simulink model "Lure_Preisach"  (R2017b)
settings: Solver=FixedStepAuto  StartTime=0.0  StopTime=simTotalTime  FixedStep=0.05  MaxStep=0.1  MinStep=0.01  RelTol=1e-3
undefined symbols (not defined in the file): gridArea, gridDen, gridLength, hysteronMax, hysteronMin, initialRelays, inputFactor, inputMax, inputMin, offset, outputFactor, outputMax, outputMin, weightFunc, xyGrid
libraries: simulink x2
settings Model: Creator=Marco  LastModifiedBy=M. Vasquez Beltran

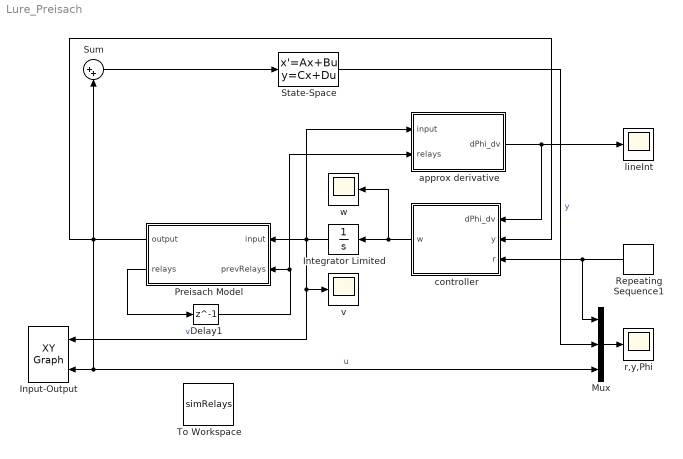
== system Lure_Preisach ==
  Delay1 : Delay  DelayLength=1  InitialCondition=initialRelays
  Input-Output : simulink/Sinks/XY Graph  xmin=inputMin*inputFactor  xmax=inputMax*inputFactor  ymin=outputMin*outputFactor  ymax=outputMax*outputFactor  st=-1
  Integrator Limited : Integrator  InitialCondition=0.75  UpperSaturationLimit=inputMax*0.99  LowerSaturationLimit=inputMin*0.99
  Mux : Mux  Inputs=3
  Preisach Model : MATLAB Function  TreatAsAtomicUnit=on
  Repeating Sequence1 : simulink/Sources/Repeating Sequence  rep_seq_t=sequenceTime  rep_seq_y=sequenceVal
  State-Space : StateSpace  A=-1  D=0  InitialCondition=-1.2
  Sum : Sum  Inputs=|++
  To Workspace : ToWorkspace  VariableName=simRelays  SampleTime=-1
  approx derivative : MATLAB Function  TreatAsAtomicUnit=on
  controller : MATLAB Function  TreatAsAtomicUnit=on
  lineInt : Scope
  r,y,Phi : Scope
  v : Scope
  w : Scope
  wires:
  Preisach Model/2(relays) -> Delay1/1
  Delay1/1 -> approx derivative/2(relays), Preisach Model/2(prevRelays)
  Sum/1 -> State-Space/1
  Preisach Model/1(output) -> controller/2(y), Sum/2, Input-Output/2, Mux/3  "u"
  State-Space/1 -> Mux/2  "y"
  Integrator Limited/1 -> approx derivative/1(input), Preisach Model/1(input), Input-Output/1, v/1  "v"
  approx derivative/1(dPhi_dv) -> controller/1(dPhi_dv), lineInt/1
  Repeating Sequence1/1 -> controller/3(r), Mux/1
  controller/1(w) -> Integrator Limited/1, w/1
  Mux/1 -> r,y,Phi/1

== matlab function Lure_Preisach/Preisach Model ==
  data: input input; prevRelays input; output output; weightFunc parameter; relays output; offset parameter; hysteronMin parameter; hysteronMax parameter; gridDen parameter; xyGrid parameter; gridLength parameter; gridArea parameter
function [output, relays] = fcn(input, prevRelays, ...
    weightFunc, offset, hysteronMin, hysteronMax, gridDen, xyGrid, gridLength, gridArea)

%     output = offset;
%     relays = prevRelays;
%     for i=1:gridDen
%         ii = gridDen-i+1; %index inversion for rows
%         for j=1:i
%             if( input >= xyGrid(i) && relays(ii,j) ~= hysteronMax )
%                 relays(ii,j) = hysteronMax;
%             elseif( input <= xyGrid(j) && relays(ii,j) ~= hysteronMin )
%                 relays(ii,j) = hysteronMin;
%             end
%             output = output + relays(ii,j)*weightFunc(ii,j)*gridArea;
%         end
%     end



%     relays = prevRelays;
%     for row=1:gridDen+1
%         if( row == gridDen+1 || input <= xyGrid(row) )
%             row = row-1;
%             irow = gridDen-row+1;
%             relays(irow:end, 1:row) = hysteronMax*fliplr(triu(ones(row, row)));
%             break;
%         end
%     end
%     for col=gridDen:-1:0
%         if( col == 0 || input >= xyGrid(col) )
%             col = col+1;
%             irow = gridDen-col+1;
%             relays(1:irow, col:end) = hysteronMin*fliplr(triu(ones(irow, irow)));
%             break;
%         end
%     end
%     output = sum(sum(relays(:,:).*weightFunc(:,:)))*gridArea + offset;



    relays = prevRelays;
    if( xyGrid(end) <= input )
        relays(:,:) = hysteronMax*fliplr(triu(ones(gridDen, gridDen)));
    elseif( input < xyGrid(1) )
        relays(:,:) = hysteronMin*fliplr(triu(ones(gridDen, gridDen)));
    else
        idx0 = 1;
        while( idx0 <= gridDen-1 )
            if( xyGrid(idx0) <= input && input < xyGrid(idx0+1) )
                col = idx0;
                row = gridDen-idx0+1;

                relays(row:end, 1:col) = hysteronMax*fliplr(triu(ones(col, col)));
                relays(1:row-1, col+1:end) = hysteronMin*fliplr(triu(ones(row-1, row-1)));
                break;
            end
            idx0 = idx0 + 1;
        end
    end
    output = sum(sum(relays(:,:).*weightFunc(:,:)))*gridArea + offset;

== matlab function Lure_Preisach/approx derivative ==
  data: input input; relays input; weightFunc parameter; hysteronMin parameter; hysteronMax parameter; offset parameter; gridDen parameter; dPhi_dv output; xyGrid parameter; gridLength parameter
function dPhi_dv = fcn(input, relays,...
     weightFunc, hysteronMin, hysteronMax, offset, gridDen, xyGrid, gridLength)

dPhi_dv = [0; 0];
if( xyGrid(end) <= input )
    return;
elseif( input < xyGrid(1) )
    return;
else
    idx0 = 1;
    while( idx0 <= gridDen-1 )
        if( xyGrid(idx0) <= input && input < xyGrid(idx0+1) )
            col = idx0;
            row = gridDen-idx0+1;
            
            for var=col:-1:1
                if( relays(row-1,var)==hysteronMin )
                    dPhi_dv(1) = dPhi_dv(1) + gridLength*weightFunc(row-1,var);
                end
            end
            
            for var=row:-1:1
                if( relays(var,col)==hysteronMax )
                    dPhi_dv(2) = dPhi_dv(2) + gridLength*weightFunc(var,col);
                end
            end
            
            break;
        end
        idx0 = idx0 + 1;
    end
end
dPhi_dv = 2*dPhi_dv;

end

== matlab function Lure_Preisach/controller ==
  data: dPhi_dv input; w output; y input; r input
function w    = fcn(dPhi_dv, y, r)

    k = 2;
    lineIntTh = 0.1;
    
%     if( abs(dPhi_dv(1)) <= lineIntTh && abs(dPhi_dv(2)) <= lineIntTh )
%         w = 0;
%     elseif( abs(dPhi_dv(1)) >= abs(dPhi_dv(2)) )
%         w = k*(r-y)/dPhi_dv(1);
%     else
%         w = -k*(r-y)/dPhi_dv(2);
%     end
    
%     w = 0;
%     signVec = dPhi_dv;
%     signVec(signVec>=0) = 1;
%     signVec(signVec<0) = -1;
%     if( abs(dPhi_dv(1)) > abs(dPhi_dv(2)) )
%         lambda = signVec(1)*max(abs([dPhi_dv(1), lineIntTh]));
%     else
%         lambda = signVec(2)*max(abs([dPhi_dv(2), lineIntTh]));
%     end
%     w = k*(r-y)/lambda;
    
    w = 0;
    if( r-y>0 )
        lambda = max(abs([dPhi_dv(1), lineIntTh]));
    else
        lambda = max(abs([dPhi_dv(2), lineIntTh]));
    end
    w = k*(r-y)/lambda;
    
%     w = 0;
%     e = r-y;
%     if ( e>0 )
%         if ( dPhi_dv(1)>0 )
%             w =  abs(e)/max(abs([lineIntTh, dPhi_dv(1)]));
%         elseif ( dPhi_dv(2)<0 )
%             w = -abs(e)/max(abs([lineIntTh, dPhi_dv(2)]));
%         elseif ( dPhi_dv(1)<=0 )
%             w = -abs(e)/max(abs([lineIntTh, dPhi_dv(2)]));
%         end
%     elseif( e<0 )
%         if ( dPhi_dv(2)>0 )
%             w = -abs(e)/max(abs([lineIntTh, dPhi_dv(2)]));
%         elseif ( dPhi_dv(1)<0 )
%             w =  abs(e)/max(abs([lineIntTh, dPhi_dv(1)]));
%         elseif ( dPhi_dv(2)<=0 )
%             w = abs(e)/max(abs([lineIntTh, dPhi_dv(1)]));
%         end
%     end
    
end
